simulink model "AngleSpeedToPWM_simu"  (R2017a)
settings: Solver=FixedStepDiscrete  StartTime=0.0  StopTime=50000  FixedStep=1  RelTol=1e-3
libraries: hdlsllib x3, simulink x1
settings Model: Creator=chandler.ga  LastModifiedBy=chandler.ga

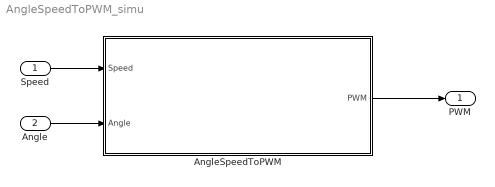
== system AngleSpeedToPWM_simu ==
  Speed : Inport
  Angle : Inport  Port=2
  AngleSpeedToPWM : Subsystem
  PWM : Outport
  wires:
  Speed/1 -> AngleSpeedToPWM/1(Speed)
  Angle/1 -> AngleSpeedToPWM/2(Angle)
  AngleSpeedToPWM/1(PWM) -> PWM/1

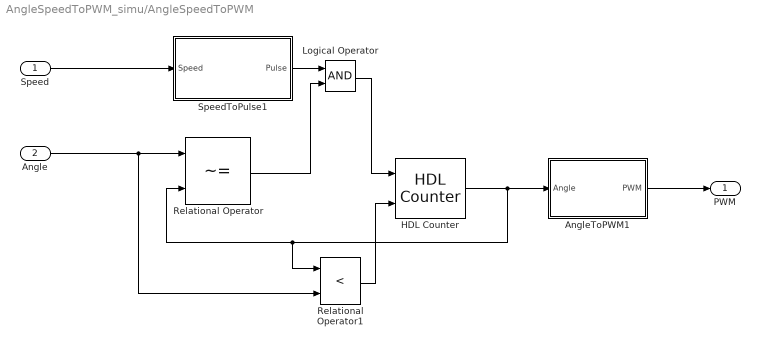
== system AngleSpeedToPWM_simu/AngleSpeedToPWM ==
  Speed : Inport
  Angle : Inport  Port=2
  AngleToPWM1 : Subsystem
  HDL Counter : hdlsllib/HDL Operations/HDL Counter  CountType=Count limited  CountInit=90  CountStep=1  CountMax=180  CountFromType=Specify  CountFrom=0  CountResetPort=off  CountLoadPort=off  CountEnbPort=on  CountDirPort=on  CountDataType=Unsigned  CountWordLen=8  CountFracLen=0  CountSampTime=1
      settings: SourceProductName=HDL Coder  SourceProductBaseCode=HD
  Logical Operator : Logic  AllPortsSameDT=off  OutDataTypeStr=boolean
  Relational Operator : RelationalOperator  Operator=~=  OutDataTypeStr=boolean  RndMeth=Simplest
  Relational Operator1 : RelationalOperator  Operator=<  OutDataTypeStr=boolean  RndMeth=Simplest
  SpeedToPulse1 : Subsystem
  PWM : Outport
  wires:
  Relational Operator1/1 -> HDL Counter/2
  Speed/1 -> SpeedToPulse1/1(Speed)
  SpeedToPulse1/1(Pulse) -> Logical Operator/1
  Angle/1 -> Relational Operator1/2, Relational Operator/1
  Relational Operator/1 -> Logical Operator/2
  Logical Operator/1 -> HDL Counter/1
  HDL Counter/1 -> AngleToPWM1/1(Angle), Relational Operator1/1, Relational Operator/2
  AngleToPWM1/1(PWM) -> PWM/1

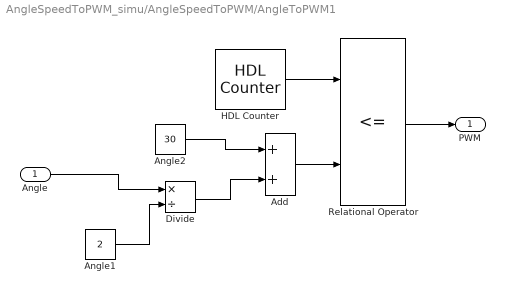
== system AngleSpeedToPWM_simu/AngleSpeedToPWM/AngleToPWM1 ==
  Angle : Inport
  Add : Sum
  Angle1 : Constant  Value=2  OutDataTypeStr=uint8
  Angle2 : Constant  Value=30  OutDataTypeStr=uint8
  Divide : Product  Inputs=*/
  HDL Counter : hdlsllib/HDL Operations/HDL Counter  CountType=Count limited  CountInit=0  CountStep=1  CountMax=1000  CountFromType=Initial value  CountFrom=0  CountResetPort=off  CountLoadPort=off  CountEnbPort=off  CountDirPort=off  CountDataType=Unsigned  CountWordLen=20  CountFracLen=0  CountSampTime=1
      settings: SourceProductName=HDL Coder  SourceProductBaseCode=HD
  Relational Operator : RelationalOperator  Operator=<=  OutDataTypeStr=boolean  RndMeth=Simplest
  PWM : Outport
  wires:
  Angle/1 -> Divide/1
  Divide/1 -> Add/2
  Relational Operator/1 -> PWM/1
  Add/1 -> Relational Operator/2
  HDL Counter/1 -> Relational Operator/1
  Angle2/1 -> Add/1
  Angle1/1 -> Divide/2

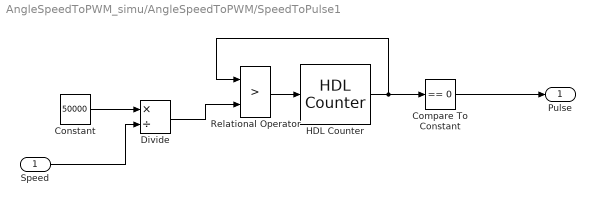
== system AngleSpeedToPWM_simu/AngleSpeedToPWM/SpeedToPulse1 ==
  Speed : Inport  OutDataTypeStr=uint8
  Compare To Constant : simulink/Logic and Bit Operations/Compare To Constant  relop===  const=0  OutDataTypeStr=boolean
  Constant : Constant  Value=50000
  Divide : Product  Inputs=*/  SaturateOnIntegerOverflow=on  RndMeth=Zero
  HDL Counter : hdlsllib/HDL Operations/HDL Counter  CountType=Free running  CountInit=0  CountStep=1  CountMax=50000000  CountFromType=Initial value  CountFrom=0  CountResetPort=on  CountLoadPort=off  CountEnbPort=off  CountDirPort=off  CountDataType=Unsigned  CountWordLen=26  CountFracLen=0  CountSampTime=1
      settings: SourceProductName=HDL Coder  SourceProductBaseCode=HD
  Relational Operator : RelationalOperator  Operator=>  OutDataTypeStr=boolean  RndMeth=Nearest
  Pulse : Outport
  wires:
  Constant/1 -> Divide/1
  HDL Counter/1 -> Relational Operator/1, Compare To Constant/1
  Divide/1 -> Relational Operator/2
  Speed/1 -> Divide/2
  Compare To Constant/1 -> Pulse/1
  Relational Operator/1 -> HDL Counter/1
